simulink model "EX1"  (R2023b)
settings: Solver=VariableStepAuto  StartTime=0.0  StopTime=3.0  RelTol=1e-3
settings Model: Creator=ousso  LastModifiedBy=ousso

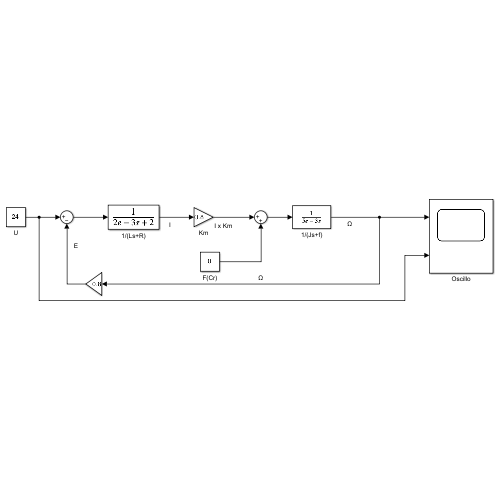
[thumbnail: Simulink's stored preview of the top-level diagram]
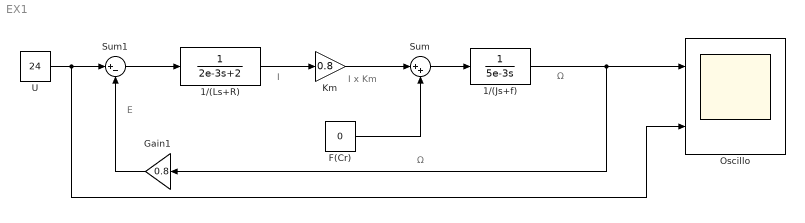
== system EX1 ==
  note: Ω
  note: I x Km
  note: I
  note: E
  note: Ω
  1/(Js+f) : TransferFcn  Denominator=[5e-3 0]
  1/(Ls+R) : TransferFcn  Denominator=[2e-3 2]
  F(Cr) : Constant  Value=0
  Gain1 : Gain  Gain=0.8
  Km : Gain  Gain=0.8
  Oscillo : Scope  NumInputPorts=2
  Sum : Sum  Inputs=|++
  Sum1 : Sum  Inputs=|+-
  U : Constant  Value=24
  wires:
  Sum1/1 -> 1/(Ls+R)/1
  1/(Ls+R)/1 -> Km/1
  Km/1 -> Sum/1
  F(Cr)/1 -> Sum/2
  Sum/1 -> 1/(Js+f)/1
  1/(Js+f)/1 -> Gain1/1, Oscillo/1
  Gain1/1 -> Sum1/2
  U/1 -> Oscillo/2, Sum1/1
